simulink model "base_band_shaping_model"  (R2020b)
settings: Solver=FixedStepDiscrete  StartTime=0.0  StopTime=400  RelTol=1e-3
libraries: dspmlti4 x2, dspmathops x1, whdlio x1, commdigbbndpm3 x1, commfilt2 x1, commrandsrc3 x1
settings Model: DataTypeOverride=Off  Creator=wardo  LastModifiedBy=EFlores
settings DataIOCC: LimitDataPoints=on  SaveOutput=off  SaveTime=off
settings OptimizationCC: BlockReduction=off  ConditionallyExecuteInputs=off  DefaultParameterBehavior=Inlined  LifeSpan=inf
settings DebuggingCC: AlgebraicLoopMsg=error  SingleTaskRateTransMsg=error  AllowSymbolicDim=off  StrictBusMsg=ErrorOnBusTreatedAsVector  SFUnexpectedBacktrackingDiag=warning  SFNoUnconditionalDefaultTransitionDiag=warning  SFExecutionAtInitializationDiag=none  ArithmeticOperatorsInVariantConditions=warning
settings HardwareCC: ProdBitPerPointer=32  ProdBitPerSizeT=32  ProdBitPerPtrDiffT=32  ProdLargestAtomicFloat=None  ProdIntDivRoundTo=Undefined  ProdEndianess=Unspecified  ProdWordSize=32  ProdHWDeviceType=ASIC/FPGA->ASIC/FPGA  ProdEqTarget=off
settings SFSimCC: SimUseLocalCustomCode=off  CustomCodeUndefinedFunction=UseInterfaceOnly
settings RTWCC: RTWUseLocalCustomCode=off
settings CodeAppCC: StateflowObjectComments=on
settings GRTTargetCC: TargetLangStandard=C89/C90 (ANSI)
settings ConfigComp: CovScope=ReferencedModels  CovMetricSettings=dw  CovSaveCumulativeToWorkspaceVar=on  CovSaveSingleToWorkspaceVar=on  CovExternalEMLEnable=off  CovSFcnEnable=off

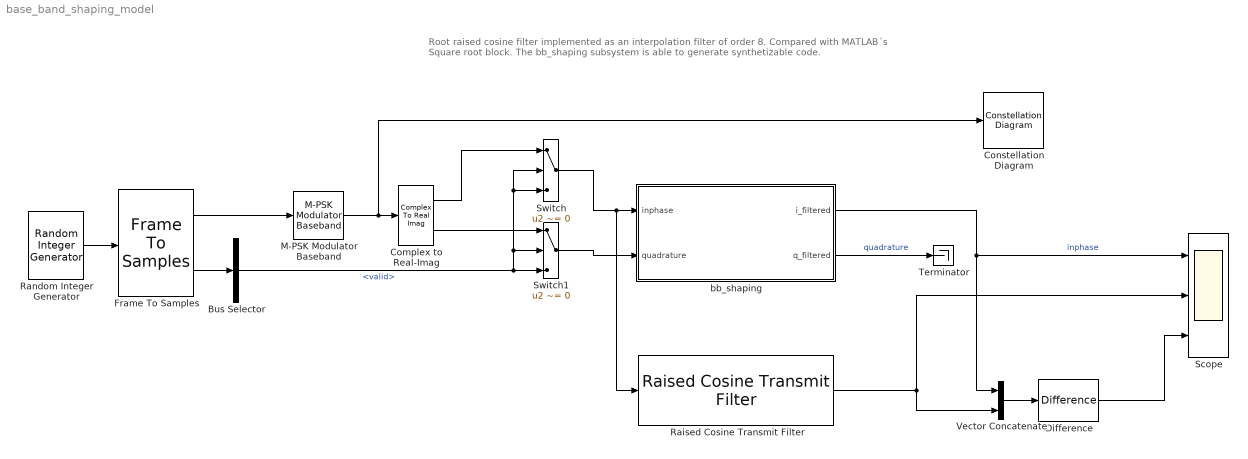
== system base_band_shaping_model ==
  note: Root raised cosine filter implemented as an interpolation filter of order 8.
      | Compared with MATLAB´s Square root block.
      |
      | The bb_shaping subsystem is able to generate synthetizable code.
  Bus Selector : BusSelector  OutputSignals=valid
  Complex to Real-Imag : ComplexToRealImag
  Constellation Diagram : ConstellationDiagram
  Difference : dspmathops/Difference  Run=No  dim=Columns  Dimension=1  roundingMode=Floor  overflowMode=off  outputDataTypeStr=Inherit: Same as accumulator  outputMin=[]  outputMax=[]  outputLastDataTypeStr=Inherit: Same as accumulator
      settings: SourceProductBaseCode=DS
  Frame To Samples : whdlio/Frame To Samples  InterSampleIdleCycles=1  InterFrameIdleCycles=100  OutputSize=1  InterleaveSamples=off
      settings: SourceProductBaseCode=LH
  M-PSK Modulator Baseband : commdigbbndpm3/M-PSK Modulator Baseband  M=8  InType=Integer  Enc=Gray  Mapping=[0:7]  Ph=0  outDtype=Fixed-point  outWordLen=18  outUDDataType=sfix(16)  outFracLenMode=User-defined  outFracLen=14  outDataTypeStr=fixdt(1,18,14)  outLastDataTypeStr=fixdt(1,18,14)
      settings: SourceProductName=Communications Toolbox
  Raised Cosine Transmit Filter : commfilt2/Raised Cosine Transmit Filter  filtType=Square root  R=0.2  filtSpan=10  N=8  filterGain=1  RateOptions=Allow multirate processing  framing=Mute  checkCoeff=off  variableName=rcTxFilt  checkGain=Normalized  sampMode=Mute  saveAsFlag=0  currentFiltSpan=10  D=5  launchFVT=on  roundingMode=Floor  overflowMode=off  coeffDataTypeStr=Inherit: Same word length as input  coeffMin=[]  coeffMax=[]  coeffLastDataTypeStr=Inherit: Same word length as input  prodOutputMode=Binary point scaling  prodOutputWordLength=34  prodOutputFracLength=30  prodOutputDataTypeStr=fixdt(1,34,30)  prodOutputLastDataTypeStr=fixdt(1,34,30)  outputDataTypeStr=Inherit: Same as accumulator  outputMin=[]  outputMax=[]  outputLastDataTypeStr=Inherit: Same as accumulator
      settings: SourceProductName=Communications Toolbox
  Random Integer Generator : commrandsrc3/Random Integer Generator  SetSize=8  SeedSource=Auto  Seed=0  SampleTime=10  SamplesPerFrame=10  OutputDataType=double  SimulateUsing=Interpreted execution
  Scope : Scope  NumInputPorts=3
  Switch : Switch  Criteria=u2 ~= 0  OutDataTypeStr=Inherit: Inherit via back propagation
  Switch1 : Switch  Criteria=u2 ~= 0  OutDataTypeStr=Inherit: Inherit via back propagation
  Terminator : Terminator
  Vector Concatenate : Concatenate
  bb_shaping : Subsystem
  wires:
  bb_shaping/1(i_filtered) -> Vector Concatenate/1, Scope/1  "inphase"
  Frame To Samples/1 -> M-PSK Modulator Baseband/1
  M-PSK Modulator Baseband/1 -> Complex to Real-Imag/1, Constellation Diagram/1
  Random Integer Generator/1 -> Frame To Samples/1
  Frame To Samples/2 -> Bus Selector/1
  Bus Selector/1 -> Switch1/3, Switch/3, Switch/2, Switch1/2  "<valid>"
  Complex to Real-Imag/1 -> Switch/1
  Switch1/1 -> bb_shaping/2(quadrature)
  Complex to Real-Imag/2 -> Switch1/1
  Switch/1 -> Raised Cosine Transmit Filter/1, bb_shaping/1(inphase)
  Raised Cosine Transmit Filter/1 -> Scope/2, Vector Concatenate/2
  Vector Concatenate/1 -> Difference/1
  Difference/1 -> Scope/3
  bb_shaping/2(q_filtered) -> Terminator/1  "quadrature"

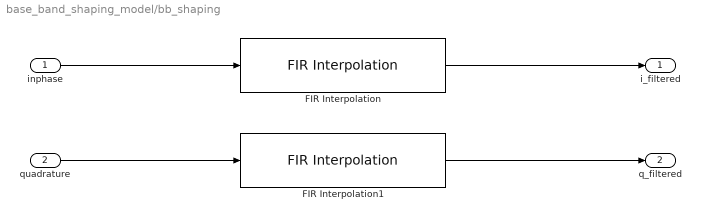
== system base_band_shaping_model/bb_shaping ==
  inphase : Inport
  quadrature : Inport  Port=2
  FIR Interpolation : dspmlti4/FIR Interpolation  FilterSource=Dialog parameters  PrivateCoeffs=0  h=[-0.00599670410156250,-0.00514221191406250,-0.00289916992187500,0.000442504882812500,0.00431823730468750,0.00794982910156250,0.0104980468750000,0.0112304687500000,0.00967407226562500,0.00578308105468750,0,-0.00680541992187500,-0.0134124755859375,-0.0184326171875000,-0.0205841064453125,-0.0189819335937500,-0.0133361816406250,-0.00410461425781250,0.00752258300781250,0.0196380615234375,0.0300140380859375,0.0363464355468750,0.0367584228515625,0.0301208496093750,0.0164794921875000,-0.00291442871093750,-0.0254821777343750,-0.0476837158203125,-0.0653228759765625,-0.0742187500000000,-0.0707244873046875,-0.0524291992187500,-0.0185852050781250,0.0296783447265625,0.0892028808593750,0.155227661132813,0.221755981445313,0.282333374023438,0.330810546875000,0.362121582031250,0.372940063476563,0.362121582031250,0.330810546875000,0.282333374023438,0.221755981445313,0.155227661132813,0.0892028808593750,0.0296783447265625,-0.0185852050781250,-0.0524291992187500,-0.0707244873046875,-0.0742187500000000,-0.0653228759765625,-0.0476837158203125,-0.0254821777343750,-0.00291442871093750,0.0164794921875000,0.0301208496093750,0.0367584228515625,0.0363464355468750,0.0300140380859375,0.0196380615234375,0.00752258300781250,-0.00410461425781250,-0.0133361816406250,-0.0189819335937500,-0.0205841064453125,-0.0184326171875000,-0.0134124755859375,-0.00680541992187500,0,0.00578308105468750,0.00967407226562500,0.0112304687500000,0.0104980468750000,0.00794982910156250,0.00431823730468750,0.000442504882812500,-0.00289916992187500,-0.00514221191406250,-0.00599670410156250]  L=8  FilterObject=FINTERP  framing=Allow multirate processing  outputBufInitCond=0  roundingMode=Floor  overflowMode=off  firstCoeffMode=Specify word length  firstCoeffWordLength=16  firstCoeffFracLength=15  firstCoeffDataTypeStr=fixdt(1,16)  firstCoeffMin=[]  firstCoeffMax=[]  firstCoeffLastDataTypeStr=fixdt(1,16)  outputDataTypeStr=Inherit: Same as accumulator  outputMin=[]  outputMax=[]  outputLastDataTypeStr=Inherit: Same as accumulator
      settings: SourceProductName=DSP System Toolbox
  FIR Interpolation1 : dspmlti4/FIR Interpolation  FilterSource=Dialog parameters  PrivateCoeffs=0  h=[-0.00599670410156250,-0.00514221191406250,-0.00289916992187500,0.000442504882812500,0.00431823730468750,0.00794982910156250,0.0104980468750000,0.0112304687500000,0.00967407226562500,0.00578308105468750,0,-0.00680541992187500,-0.0134124755859375,-0.0184326171875000,-0.0205841064453125,-0.0189819335937500,-0.0133361816406250,-0.00410461425781250,0.00752258300781250,0.0196380615234375,0.0300140380859375,0.0363464355468750,0.0367584228515625,0.0301208496093750,0.0164794921875000,-0.00291442871093750,-0.0254821777343750,-0.0476837158203125,-0.0653228759765625,-0.0742187500000000,-0.0707244873046875,-0.0524291992187500,-0.0185852050781250,0.0296783447265625,0.0892028808593750,0.155227661132813,0.221755981445313,0.282333374023438,0.330810546875000,0.362121582031250,0.372940063476563,0.362121582031250,0.330810546875000,0.282333374023438,0.221755981445313,0.155227661132813,0.0892028808593750,0.0296783447265625,-0.0185852050781250,-0.0524291992187500,-0.0707244873046875,-0.0742187500000000,-0.0653228759765625,-0.0476837158203125,-0.0254821777343750,-0.00291442871093750,0.0164794921875000,0.0301208496093750,0.0367584228515625,0.0363464355468750,0.0300140380859375,0.0196380615234375,0.00752258300781250,-0.00410461425781250,-0.0133361816406250,-0.0189819335937500,-0.0205841064453125,-0.0184326171875000,-0.0134124755859375,-0.00680541992187500,0,0.00578308105468750,0.00967407226562500,0.0112304687500000,0.0104980468750000,0.00794982910156250,0.00431823730468750,0.000442504882812500,-0.00289916992187500,-0.00514221191406250,-0.00599670410156250]  L=8  FilterObject=FINTERP  framing=Allow multirate processing  outputBufInitCond=0  roundingMode=Floor  overflowMode=off  firstCoeffMode=Specify word length  firstCoeffWordLength=16  firstCoeffFracLength=15  firstCoeffDataTypeStr=fixdt(1,16)  firstCoeffMin=[]  firstCoeffMax=[]  firstCoeffLastDataTypeStr=fixdt(1,16)  outputDataTypeStr=Inherit: Same as accumulator  outputMin=[]  outputMax=[]  outputLastDataTypeStr=Inherit: Same as accumulator
      settings: SourceProductName=DSP System Toolbox
  i_filtered : Outport  VectorParamsAs1DForOutWhenUnconnected=off
  q_filtered : Outport  Port=2  VectorParamsAs1DForOutWhenUnconnected=off
  wires:
  inphase/1 -> FIR Interpolation/1
  FIR Interpolation/1 -> i_filtered/1
  FIR Interpolation1/1 -> q_filtered/1
  quadrature/1 -> FIR Interpolation1/1
